simulink model "PMSM_Lq_Ke"  (R2024a)
settings: Solver=FixedStepAuto  StartTime=0.0  StopTime=0.5  FixedStep=1E-6  RelTol=1e-3
model workspace (MAT data in the model file):
  PWM_Frequency = Simulink.Parameter
  PWM_Frequency.Value = 30000
  PWM_Frequency.Complexity = 'real'
  PWM_Frequency.Dimensions = [1 1]
  PWM_Frequency.DataType = 'double'
  TimerPeriod = 0.1
values from neighbouring files (symbols this model uses):
  Flux = 0.01837    [Flux_Nonsensor_data_new.m]
undefined symbols (not defined in the file or in its folder): Down, Up
libraries: eePwmGenerator x4, slpidlib x3, spsDCVoltageSourceLib x1, spsPermanentMagnetSynchronousMachineLib x1, spsUniversalBridgeLib x1, sps_lib x1
settings Model: Creator=shish  LastModifiedBy=shish

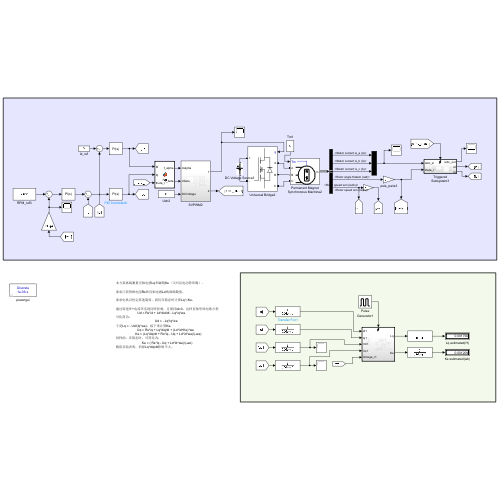
[thumbnail: Simulink's stored preview of the top-level diagram]
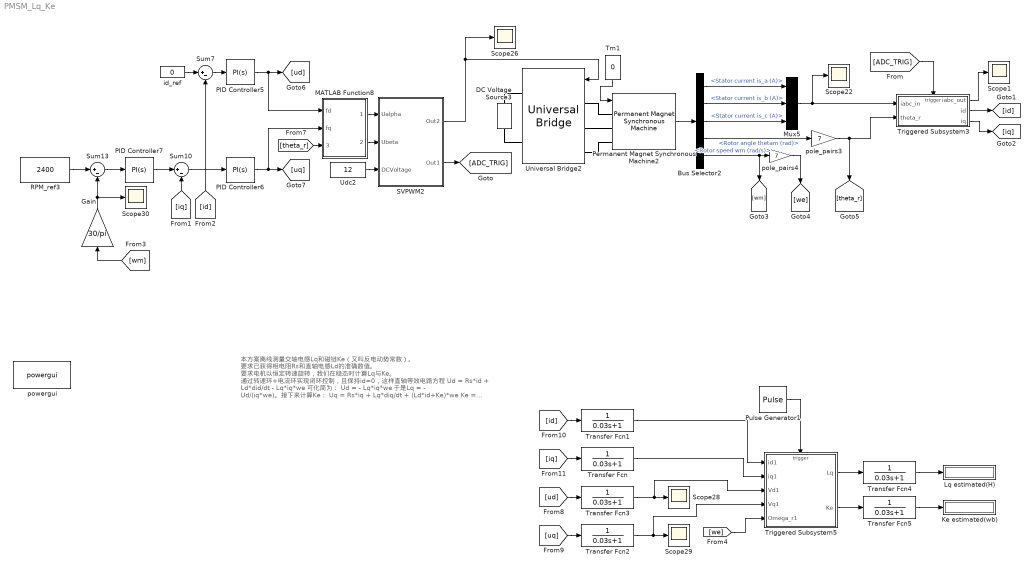
== system PMSM_Lq_Ke ==
  note: 本方案离线测量交轴电感Lq和磁链Ke（又叫反电动势常数）。
      |
      | 要求已获得相电阻Rs和直轴电感Ld的准确数值。
      |
      | 要求电机以恒定转速旋转，我们在稳态时计算Lq与Ke。
      |
      | 通过转速环+电流环实现闭环控制，且保持id=0，这样直轴等效电路方程
      |                         Ud = Rs*id + Ld*did/dt - Lq*iq*we
      | 可化简为：
      | 						Ud = - Lq*iq*we
      | 于是Lq = - Ud/(iq*we)。接下来计算Ke：
      | 			  Uq = Rs*iq + Lq*diq/dt + (Ld*id+Ke)*we
      | 			Ke = (Lq*diq/dt + Rs*iq - Uq + Ld*id*we)/(-we)
      | 同样的，在稳态时，可简化为：
      | 				Ke = ( Rs*iq - Uq + Ld*id*we)/(-we)
      | 数值实验表明，扔掉Lq*diq/dt影响不大。
  Bus Selector2 : BusSelector  OutputSignals=Stator current is_a (A),Stator current is_b (A),Stator current is_c (A),Rotor angle thetam (rad),Rotor speed wm (rad/s)
  DC Voltage Source3 : spsDCVoltageSourceLib/DC Voltage Source  Amplitude=12  Measurements=Voltage
  Gain : Gain  Gain=30/pi
  Ke estimated(wb) : Display
  Lq estimated(H) : Display
  MATLAB Function8 : MATLAB Function  TreatAsAtomicUnit=on
  Mux5 : Mux  Inputs=3
  PID Controller5 : slpidlib/PID Controller  Controller=PI  Form=Parallel  TimeDomain=Continuous-time  UseExternalTs=off  SampleTime=-1  IntegratorMethod=Forward Euler  FilterMethod=Forward Euler  ControllerParametersSource=internal  P=5  I=1  UseKiTs=on  D=0  UseExternalDerivativeSource=off  N=100  UseFilter=on  TunerSelectOption=Transfer Function Based (PID Tuner App)  InitialConditionSource=internal  InitialConditionForIntegrator=0  InitialConditionForFilter=0  DifferentiatorICPrevScaledInput=0  ExternalReset=none  TrackingMode=off  Kt=1  LimitOutput=off  SatLimitsSource=internal  UpperSaturationLimit=inf  LowerSaturationLimit=-inf  LinearizeAsGain=on  AntiWindupMode=none  Kb=1  LimitIntegrator=off  UpperIntegratorSaturationLimit=inf  LowerIntegratorSaturationLimit=-inf  POutMin=[]  POutMax=[]  IOutMin=[]  IOutMax=[]  DOutMin=[]  DOutMax=[]  NOutMin=[]  NOutMax=[]  SumOutMin=[]  SumOutMax=[]  SaturationOutMin=[]  SaturationOutMax=[]  PParamMin=[]  PParamMax=[]  IParamMin=[]  IParamMax=[]  DParamMin=[]  DParamMax=[]  NParamMin=[]  NParamMax=[]  KbParamMin=[]  KbParamMax=[]  KtParamMin=[]  KtParamMax=[]  KbOutMin=[]  KbOutMax=[]  KtOutMin=[]  KtOutMax=[]  IntegratorOutMin=[]  IntegratorOutMax=[]  FilterOutMin=[]  FilterOutMax=[]  SumI1OutMin=[]  SumI1OutMax=[]  SumI2OutMin=[]  SumI2OutMax=[]  SumI3OutMin=[]  SumI3OutMax=[]  SumI4OutMin=[]  SumI4OutMax=[]  SumDOutMin=[]  SumDOutMax=[]  DifferentiatorOutMin=[]  DifferentiatorOutMax=[]  FilterDiffOutCoefMin=[]  FilterDiffOutCoefMax=[]  ReciprocalOutMin=[]  ReciprocalOutMax=[]  SumDenOutMin=[]  SumDenOutMax=[]  SumNumOutMin=[]  SumNumOutMax=[]  DivideOutMin=[]  DivideOutMax=[]  UdiffTsProdOutMin=[]  UdiffTsProdOutMax=[]  NTsProdOutMin=[]  NTsProdOutMax=[]  UintegralTsProdOutMin=[]  UintegralTsProdOutMax=[]  UngainTsProdOutMin=[]  UngainTsProdOutMax=[]  ClampingZeroOutDataTypeStr=Inherit: Inherit via back propagation  ClampingZeroOutMin=[]  ClampingZeroOutMax=[]  FilterDenConstantOutDataTypeStr=Inherit: Inherit via back propagation  FilterDenConstantOutMin=[]  FilterDenConstantOutMax=[]  PCopyOutDataTypeStr=Inherit: Inherit via back propagation  PCopyOutMin=[]  PCopyOutMax=[]  NCopyOutDataTypeStr=Inherit: Inherit via back propagation  NCopyOutMin=[]  NCopyOutMax=[]  IntegratorContinuousStateAttributes=''  IntegratorStateMustResolveToSignalObject=off  IntegratorRTWStateStorageClass=Auto  FilterContinuousStateAttributes=''  FilterStateMustResolveToSignalObject=off  FilterRTWStateStorageClass=Auto  ParallelPVariant=InternalParameters  IdealPVariant=Disabled  IVariant=InternalParameters  DVariant=Disabled  IntegratorVariant=Continuous  SatVariant=Disabled  AWVariant=Passthrough  PCopyVariant=Disabled  TRVariant=Disabled  FdbkBlocksVariant=Forward  IdealPFdbkVariant=Disabled  SatFdbkVariant=Disabled  DerivativeFilterVariant=Disabled  NVariant=Disabled  NCopyVariant=Disabled_SignalSpec  FilterICVariant=Disabled  IntegratorICVariant=InternalICs  ExternalResetVariant=Disabled  TRSumVariant=Passthrough  SumFdbkVariant=Disabled  SumVariant=Sum_PI  TsampFilterVariant=InternalTs  TsampNgainVariant=Passthrough  TsampIntegralVariant=Disabled_SignalSpec  ExternalSaturationOutDataTypeStr=Inherit: Same as second input  DerivativeSourceVariant=Disabled
  PID Controller6 : slpidlib/PID Controller  Controller=PI  Form=Parallel  TimeDomain=Continuous-time  UseExternalTs=off  SampleTime=-1  IntegratorMethod=Forward Euler  FilterMethod=Forward Euler  ControllerParametersSource=internal  P=5  I=1  UseKiTs=on  D=0  UseExternalDerivativeSource=off  N=100  UseFilter=on  TunerSelectOption=Transfer Function Based (PID Tuner App)  InitialConditionSource=internal  InitialConditionForIntegrator=0  InitialConditionForFilter=0  DifferentiatorICPrevScaledInput=0  ExternalReset=none  TrackingMode=off  Kt=1  LimitOutput=off  SatLimitsSource=internal  UpperSaturationLimit=inf  LowerSaturationLimit=-inf  LinearizeAsGain=on  AntiWindupMode=none  Kb=1  LimitIntegrator=off  UpperIntegratorSaturationLimit=inf  LowerIntegratorSaturationLimit=-inf  POutMin=[]  POutMax=[]  IOutMin=[]  IOutMax=[]  DOutMin=[]  DOutMax=[]  NOutMin=[]  NOutMax=[]  SumOutMin=[]  SumOutMax=[]  SaturationOutMin=[]  SaturationOutMax=[]  PParamMin=[]  PParamMax=[]  IParamMin=[]  IParamMax=[]  DParamMin=[]  DParamMax=[]  NParamMin=[]  NParamMax=[]  KbParamMin=[]  KbParamMax=[]  KtParamMin=[]  KtParamMax=[]  KbOutMin=[]  KbOutMax=[]  KtOutMin=[]  KtOutMax=[]  IntegratorOutMin=[]  IntegratorOutMax=[]  FilterOutMin=[]  FilterOutMax=[]  SumI1OutMin=[]  SumI1OutMax=[]  SumI2OutMin=[]  SumI2OutMax=[]  SumI3OutMin=[]  SumI3OutMax=[]  SumI4OutMin=[]  SumI4OutMax=[]  SumDOutMin=[]  SumDOutMax=[]  DifferentiatorOutMin=[]  DifferentiatorOutMax=[]  FilterDiffOutCoefMin=[]  FilterDiffOutCoefMax=[]  ReciprocalOutMin=[]  ReciprocalOutMax=[]  SumDenOutMin=[]  SumDenOutMax=[]  SumNumOutMin=[]  SumNumOutMax=[]  DivideOutMin=[]  DivideOutMax=[]  UdiffTsProdOutMin=[]  UdiffTsProdOutMax=[]  NTsProdOutMin=[]  NTsProdOutMax=[]  UintegralTsProdOutMin=[]  UintegralTsProdOutMax=[]  UngainTsProdOutMin=[]  UngainTsProdOutMax=[]  ClampingZeroOutDataTypeStr=Inherit: Inherit via back propagation  ClampingZeroOutMin=[]  ClampingZeroOutMax=[]  FilterDenConstantOutDataTypeStr=Inherit: Inherit via back propagation  FilterDenConstantOutMin=[]  FilterDenConstantOutMax=[]  PCopyOutDataTypeStr=Inherit: Inherit via back propagation  PCopyOutMin=[]  PCopyOutMax=[]  NCopyOutDataTypeStr=Inherit: Inherit via back propagation  NCopyOutMin=[]  NCopyOutMax=[]  IntegratorContinuousStateAttributes=''  IntegratorStateMustResolveToSignalObject=off  IntegratorRTWStateStorageClass=Auto  FilterContinuousStateAttributes=''  FilterStateMustResolveToSignalObject=off  FilterRTWStateStorageClass=Auto  ParallelPVariant=InternalParameters  IdealPVariant=Disabled  IVariant=InternalParameters  DVariant=Disabled  IntegratorVariant=Continuous  SatVariant=Disabled  AWVariant=Passthrough  PCopyVariant=Disabled  TRVariant=Disabled  FdbkBlocksVariant=Forward  IdealPFdbkVariant=Disabled  SatFdbkVariant=Disabled  DerivativeFilterVariant=Disabled  NVariant=Disabled  NCopyVariant=Disabled_SignalSpec  FilterICVariant=Disabled  IntegratorICVariant=InternalICs  ExternalResetVariant=Disabled  TRSumVariant=Passthrough  SumFdbkVariant=Disabled  SumVariant=Sum_PI  TsampFilterVariant=InternalTs  TsampNgainVariant=Passthrough  TsampIntegralVariant=Disabled_SignalSpec  ExternalSaturationOutDataTypeStr=Inherit: Same as second input  DerivativeSourceVariant=Disabled
  PID Controller7 : slpidlib/PID Controller  Controller=PI  Form=Parallel  TimeDomain=Continuous-time  UseExternalTs=off  SampleTime=-1  IntegratorMethod=Forward Euler  FilterMethod=Forward Euler  ControllerParametersSource=internal  P=0.008  I=0.005  UseKiTs=on  D=0  UseExternalDerivativeSource=off  N=100  UseFilter=on  TunerSelectOption=Transfer Function Based (PID Tuner App)  InitialConditionSource=internal  InitialConditionForIntegrator=0  InitialConditionForFilter=0  DifferentiatorICPrevScaledInput=0  ExternalReset=none  TrackingMode=off  Kt=1  LimitOutput=off  SatLimitsSource=internal  UpperSaturationLimit=inf  LowerSaturationLimit=-inf  LinearizeAsGain=on  AntiWindupMode=none  Kb=1  LimitIntegrator=off  UpperIntegratorSaturationLimit=inf  LowerIntegratorSaturationLimit=-inf  POutMin=[]  POutMax=[]  IOutMin=[]  IOutMax=[]  DOutMin=[]  DOutMax=[]  NOutMin=[]  NOutMax=[]  SumOutMin=[]  SumOutMax=[]  SaturationOutMin=[]  SaturationOutMax=[]  PParamMin=[]  PParamMax=[]  IParamMin=[]  IParamMax=[]  DParamMin=[]  DParamMax=[]  NParamMin=[]  NParamMax=[]  KbParamMin=[]  KbParamMax=[]  KtParamMin=[]  KtParamMax=[]  KbOutMin=[]  KbOutMax=[]  KtOutMin=[]  KtOutMax=[]  IntegratorOutMin=[]  IntegratorOutMax=[]  FilterOutMin=[]  FilterOutMax=[]  SumI1OutMin=[]  SumI1OutMax=[]  SumI2OutMin=[]  SumI2OutMax=[]  SumI3OutMin=[]  SumI3OutMax=[]  SumI4OutMin=[]  SumI4OutMax=[]  SumDOutMin=[]  SumDOutMax=[]  DifferentiatorOutMin=[]  DifferentiatorOutMax=[]  FilterDiffOutCoefMin=[]  FilterDiffOutCoefMax=[]  ReciprocalOutMin=[]  ReciprocalOutMax=[]  SumDenOutMin=[]  SumDenOutMax=[]  SumNumOutMin=[]  SumNumOutMax=[]  DivideOutMin=[]  DivideOutMax=[]  UdiffTsProdOutMin=[]  UdiffTsProdOutMax=[]  NTsProdOutMin=[]  NTsProdOutMax=[]  UintegralTsProdOutMin=[]  UintegralTsProdOutMax=[]  UngainTsProdOutMin=[]  UngainTsProdOutMax=[]  ClampingZeroOutDataTypeStr=Inherit: Inherit via back propagation  ClampingZeroOutMin=[]  ClampingZeroOutMax=[]  FilterDenConstantOutDataTypeStr=Inherit: Inherit via back propagation  FilterDenConstantOutMin=[]  FilterDenConstantOutMax=[]  PCopyOutDataTypeStr=Inherit: Inherit via back propagation  PCopyOutMin=[]  PCopyOutMax=[]  NCopyOutDataTypeStr=Inherit: Inherit via back propagation  NCopyOutMin=[]  NCopyOutMax=[]  IntegratorContinuousStateAttributes=''  IntegratorStateMustResolveToSignalObject=off  IntegratorRTWStateStorageClass=Auto  FilterContinuousStateAttributes=''  FilterStateMustResolveToSignalObject=off  FilterRTWStateStorageClass=Auto  ParallelPVariant=InternalParameters  IdealPVariant=Disabled  IVariant=InternalParameters  DVariant=Disabled  IntegratorVariant=Continuous  SatVariant=Disabled  AWVariant=Passthrough  PCopyVariant=Disabled  TRVariant=Disabled  FdbkBlocksVariant=Forward  IdealPFdbkVariant=Disabled  SatFdbkVariant=Disabled  DerivativeFilterVariant=Disabled  NVariant=Disabled  NCopyVariant=Disabled_SignalSpec  FilterICVariant=Disabled  IntegratorICVariant=InternalICs  ExternalResetVariant=Disabled  TRSumVariant=Passthrough  SumFdbkVariant=Disabled  SumVariant=Sum_PI  TsampFilterVariant=InternalTs  TsampNgainVariant=Passthrough  TsampIntegralVariant=Disabled_SignalSpec  ExternalSaturationOutDataTypeStr=Inherit: Same as second input  DerivativeSourceVariant=Disabled
  Permanent Magnet Synchronous Machine2 : spsPermanentMagnetSynchronousMachineLib/Permanent Magnet Synchronous Machine  NbPhases=3  FluxDistribution=Sinusoidal  RotorType=Salient-pole  MechanicalLoad=Torque Tm  PresetModel=No  ShowDetailedParameters=on  MeasurementBus=off  Resistance=0.05  Inductance=8.5e-3  dqInductances=[1.8e-3,1.75e-3]  La=0.000395  MachineConstant=Flux linkage established by magnets (V.s)  Flux=0.0012  VoltageCst=1.5236  TorqueCst=0.0126  Flat=120  Mechanical=[0.000012 0.000005 7 0]  PolePairs=4  InitialConditions=[0,0, 0,0]  InitialConditions5ph=[0 0 0 0 0 0]  RefAngle=Aligned with phase A axis (original Park)  IterativeDiscreteModel=Trapezoidal non iterative  TsBlock=-1  TsPowergui=0
  Pulse Generator1 : DiscretePulseGenerator  PulseType=Time based  Period=0.005  PulseWidth=30
  RPM_ref3 : Constant  Value=2400
  SVPWM2 : Subsystem
  Scope{1,22,26,28..30} (6 alike) : Scope
  Sum10 : Sum  Inputs=|+-
  Sum13 : Sum  Inputs=|+-
  Sum7 : Sum  Inputs=|+-
  Tm1 : Constant  Value=0
  Transfer Fcn{,1..5} (6 alike) : TransferFcn  Denominator=[0.03 1]
  Triggered Subsystem3 : Subsystem  TreatAsAtomicUnit=on
  Triggered Subsystem5 : Subsystem  TreatAsAtomicUnit=on
  Udc2 : Constant  Value=12
  Universal Bridge2 : spsUniversalBridgeLib/Universal Bridge  Arms=3  SnubberResistance=1e5  SnubberCapacitance=inf  Device=MOSFET / Diodes  Ron=1e-3  Lon=0  ForwardVoltages="[  0  0  ]"  ForwardVoltage=0  GTOparameters=[ 10e-6 , 20e-6 ]  IGBTparameters=[ 1e-6 , 2e-6 ]  Measurements=None  Measurements_2=None  converterType=Rectifier
  id_ref : Constant  Value=0
  pole_pairs3 : Gain  Gain=7
  pole_pairs4 : Gain  Gain=7
  powergui : sps_lib/powergui  Priority=1  SimulationMode=Discrete  SampleTime=1e-6  frequency=60  Iterations=50  frequencyindice=0  Pbase=100e6  ErrMax=1e-4  UnitsV=kV  UnitsW=MW  buscounter=0  FunctionMessages=off  echomessages=off  EnableUseOfTLC=off  CurrentSourceSwitches=off  DisableSnubberDevices=off  DisableRonSwitches=off  DisableVfSwitches=off  DisplayEquations=off  AutomaticDiscreteSolvers=off  SolverType=Tustin/Backward Euler (TBE)  Interpol=off  ExternalGateDelay=off  methode=off  Ts=100  x0status=blocks  SPID=on  SwTol=0  HookPort=off  NonlinearTolerance=1e-4  nMaxIteration=100  ContinueOnMaxIteration=off  RestoreLinks=warning  ResistiveCurrentMeasurement=off  Frange=[0:2:500]  Ylog=off  Xlog=on  ShowGrid=off  save=off  variable=ZData  structure=0  ZoomFFT=off  StartTime=0.0  cycles=1  DisplayStyle=1  fundamental=60  FreqAxis=off  MaxFrequency=1000  frequencyindicesteady=1  RmsSteady=1  display=off
  wires:
  Bus Selector2/5 -> pole_pairs4/1, [wm]  "<Rotor speed wm (rad/s)>"
  MATLAB Function8/2(f_beta) -> SVPWM2/2(Ubeta)
  Bus Selector2/3 -> Mux5/3  "<Stator current is_c (A)>"
  MATLAB Function8/1(f_alpha) -> SVPWM2/1(Ualpha)
  Permanent Magnet Synchronous Machine2/1 -> Bus Selector2/1
  Bus Selector2/4 -> pole_pairs3/1  "<Rotor angle thetam (rad)>"
  Udc2/1 -> SVPWM2/3(DCVoltage)
  Bus Selector2/2 -> Mux5/2  "<Stator current is_b (A)>"
  Sum7/1 -> PID Controller5/1
  Sum10/1 -> PID Controller6/1
  PID Controller6/1 -> [uq], MATLAB Function8/2(fq)
  Mux5/1 -> Triggered Subsystem3/1(iabc_in), Scope22/1
  Tm1/1 -> Permanent Magnet Synchronous Machine2/1
  SVPWM2/1(Out2) -> Scope26/1, Universal Bridge2/1
  Bus Selector2/1 -> Mux5/1  "<Stator current is_a (A)>"
  id_ref/1 -> Sum7/1
  PID Controller5/1 -> [ud], MATLAB Function8/1(fd)
  Triggered Subsystem3/2(id) -> [id]
  Triggered Subsystem3/3(iq) -> [iq]
  pole_pairs4/1 -> [we]
  Transfer Fcn3/1 -> Triggered Subsystem5/3(Vd1), Scope28/1
  Transfer Fcn2/1 -> Triggered Subsystem5/4(Vq1), Scope29/1
  Gain/1 -> Scope30/1, Sum13/2
  Sum13/1 -> PID Controller7/1
  PID Controller7/1 -> Sum10/1
  Pulse Generator1/1 -> Triggered Subsystem5/Trigger
  SVPWM2/2(Out1) -> [ADC_TRIG]
  [ADC_TRIG] -> Triggered Subsystem3/Trigger
  [iq] -> Sum10/2
  [id] -> Sum7/2
  [wm] -> Gain/1
  [we] -> Triggered Subsystem5/5(Omega_r1)
  pole_pairs3/1 -> Triggered Subsystem3/2(theta_r), [theta_r]
  [theta_r] -> MATLAB Function8/3(theta_r)
  [ud] -> Transfer Fcn3/1
  [uq] -> Transfer Fcn2/1
  [id] -> Transfer Fcn1/1
  [iq] -> Transfer Fcn/1
  Transfer Fcn/1 -> Triggered Subsystem5/2(iq1)
  Transfer Fcn1/1 -> Triggered Subsystem5/1(id1)
  RPM_ref3/1 -> Sum13/1
  Triggered Subsystem5/1(Lq) -> Transfer Fcn4/1
  Triggered Subsystem5/2(Ke) -> Transfer Fcn5/1
  Transfer Fcn4/1 -> Lq estimated(H)/1
  Transfer Fcn5/1 -> Ke estimated(wb)/1
  Triggered Subsystem3/1(iabc_out) -> Scope1/1
  connections:
  Universal Bridge2/LConn2 -- Permanent Magnet Synchronous Machine2/LConn2
  Universal Bridge2/LConn1 -- Permanent Magnet Synchronous Machine2/LConn1
  DC Voltage Source3/LConn1 -- Universal Bridge2/RConn2
  DC Voltage Source3/RConn1 -- Universal Bridge2/RConn1
  Universal Bridge2/LConn3 -- Permanent Magnet Synchronous Machine2/LConn3

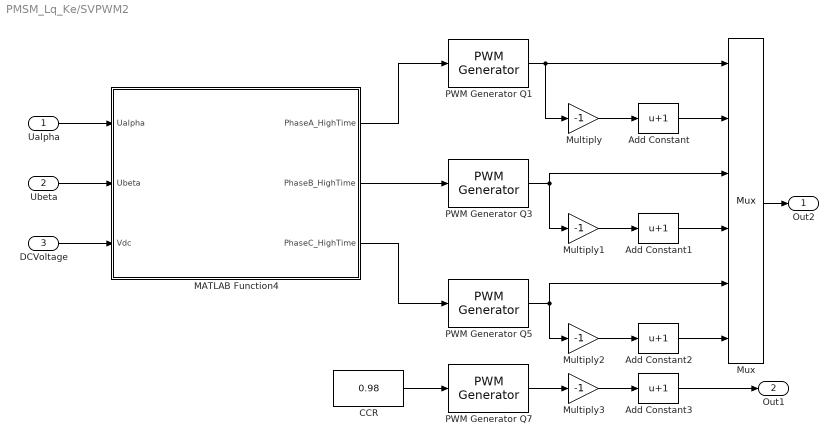
== system PMSM_Lq_Ke/SVPWM2 ==
  Ualpha : Inport
  Ubeta : Inport  Port=2
  DCVoltage : Inport  Port=3
  Add Constant{,1..3} (4 alike) : Bias  Bias=1  SaturateOnIntegerOverflow=off
  CCR : Constant  Value=0.98
  MATLAB Function4 : MATLAB Function  TreatAsAtomicUnit=on
  Multiply{,1..3} (4 alike) : Gain  Gain=-1
  Mux : Mux  Inputs=6
  PWM Generator Q{1,3,5,7} (4 alike) : eePwmGenerator/PWM Generator  CarrCount=Up-Down  Tper=1.0/PWM_Frequency  Tdelay=0  Ts=1E-6
  Out2 : Outport
  Out1 : Outport  Port=2
  wires:
  PWM Generator Q5/1 -> Mux/5, Multiply2/1
  PWM Generator Q1/1 -> Multiply/1, Mux/1
  Add Constant1/1 -> Mux/4
  Ubeta/1 -> MATLAB Function4/2(Ubeta)
  DCVoltage/1 -> MATLAB Function4/3(Vdc)
  MATLAB Function4/3(PhaseC_HighTime) -> PWM Generator Q5/1
  Multiply/1 -> Add Constant/1
  Multiply2/1 -> Add Constant2/1
  Add Constant/1 -> Mux/2
  MATLAB Function4/2(PhaseB_HighTime) -> PWM Generator Q3/1
  Add Constant2/1 -> Mux/6
  Multiply1/1 -> Add Constant1/1
  MATLAB Function4/1(PhaseA_HighTime) -> PWM Generator Q1/1
  Ualpha/1 -> MATLAB Function4/1(Ualpha)
  PWM Generator Q3/1 -> Mux/3, Multiply1/1
  PWM Generator Q7/1 -> Multiply3/1
  CCR/1 -> PWM Generator Q7/1
  Multiply3/1 -> Add Constant3/1
  Add Constant3/1 -> Out1/1
  Mux/1 -> Out2/1

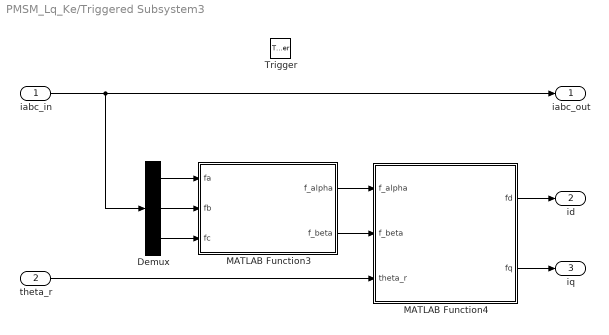
== system PMSM_Lq_Ke/Triggered Subsystem3 ==
  iabc_in : Inport
  theta_r : Inport  Port=2
  Trigger : TriggerPort  VariantControl=(inherit)
  Demux : Demux  Outputs=3
  MATLAB Function3 : MATLAB Function  TreatAsAtomicUnit=on
  MATLAB Function4 : MATLAB Function  TreatAsAtomicUnit=on
  iabc_out : Outport
  id : Outport  Port=2
  iq : Outport  Port=3
  wires:
  iabc_in/1 -> Demux/1, iabc_out/1
  Demux/3 -> MATLAB Function3/3(fc)
  Demux/2 -> MATLAB Function3/2(fb)
  Demux/1 -> MATLAB Function3/1(fa)
  MATLAB Function3/1(f_alpha) -> MATLAB Function4/1(f_alpha)
  MATLAB Function3/2(f_beta) -> MATLAB Function4/2(f_beta)
  theta_r/1 -> MATLAB Function4/3(theta_r)
  MATLAB Function4/1(fd) -> id/1
  MATLAB Function4/2(fq) -> iq/1

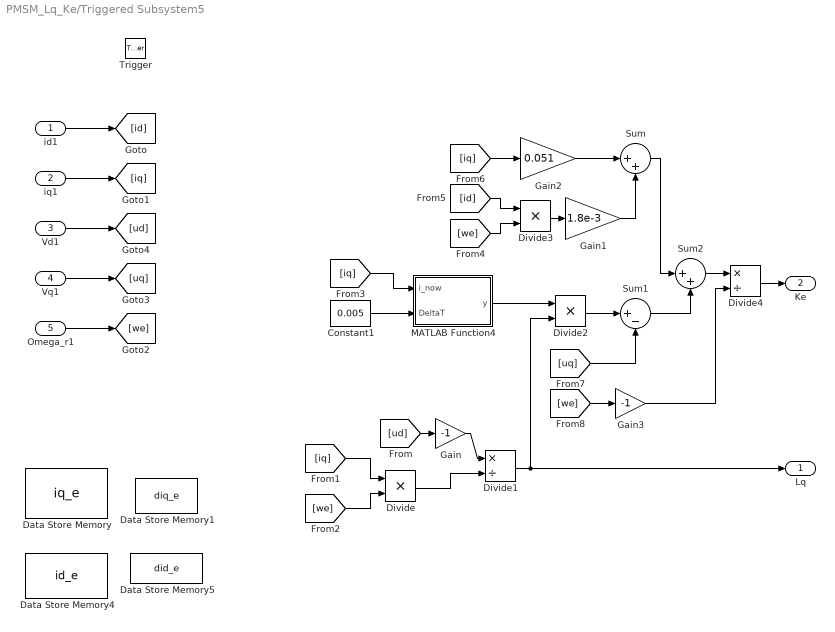
== system PMSM_Lq_Ke/Triggered Subsystem5 ==
  id1 : Inport
  iq1 : Inport  Port=2
  Vd1 : Inport  Port=3
  Vq1 : Inport  Port=4
  Omega_r1 : Inport  Port=5
  Trigger : TriggerPort  VariantControl=(inherit)
  Constant1 : Constant  Value=0.005
  Data Store Memory : DataStoreMemory  DataStoreName=iq_e  WriteAfterWriteMsg=warning  ShowAdditionalParam=off  OutDataTypeStr=double
  Data Store Memory1 : DataStoreMemory  DataStoreName=diq_e  WriteAfterWriteMsg=warning  ShowAdditionalParam=off  OutDataTypeStr=double
  Data Store Memory4 : DataStoreMemory  DataStoreName=id_e  WriteAfterWriteMsg=warning  ShowAdditionalParam=off  OutDataTypeStr=double
  Data Store Memory5 : DataStoreMemory  DataStoreName=did_e  WriteAfterWriteMsg=warning  ShowAdditionalParam=off  OutDataTypeStr=double
  Divide : Product  Inputs=**
  Divide1 : Product  Inputs=*/
  Divide2 : Product  Inputs=**
  Divide3 : Product  Inputs=**
  Divide4 : Product  Inputs=*/
  Gain : Gain  Gain=-1
  Gain1 : Gain  Gain=1.8e-3
  Gain2 : Gain  Gain=0.051
  Gain3 : Gain  Gain=-1
  MATLAB Function4 : MATLAB Function  TreatAsAtomicUnit=on
  Sum : Sum  Inputs=|++
  Sum1 : Sum  Inputs=|+-
  Sum2 : Sum  Inputs=|++
  Lq : Outport
  Ke : Outport  Port=2
  wires:
  Vd1/1 -> [ud]
  Vq1/1 -> [uq]
  Omega_r1/1 -> [we]
  id1/1 -> [id]
  iq1/1 -> [iq]
  Gain/1 -> Divide1/1
  Divide/1 -> Divide1/2
  Divide1/1 -> Divide2/2, Lq/1
  [ud] -> Gain/1
  [iq] -> Divide/1
  [we] -> Divide/2
  [iq] -> MATLAB Function4/1(i_now)
  Constant1/1 -> MATLAB Function4/2(DeltaT)
  MATLAB Function4/1(y) -> Divide2/1
  [id] -> Divide3/1
  [we] -> Divide3/2
  Divide3/1 -> Gain1/1
  [iq] -> Gain2/1
  Gain2/1 -> Sum/1
  Gain1/1 -> Sum/2
  [uq] -> Sum1/2
  Sum/1 -> Sum2/1
  Sum1/1 -> Sum2/2
  Sum2/1 -> Divide4/1
  Divide4/1 -> Ke/1
  [we] -> Gain3/1
  Gain3/1 -> Divide4/2
  Divide2/1 -> Sum1/1

== matlab function PMSM_Lq_Ke/Triggered Subsystem5/MATLAB Function4 ==
  data: i_now input; y output; iq_e data_store_memory; diq_e data_store_memory; DeltaT input
function y = TD(i_now,DeltaT)
	global iq_e;
    global diq_e;
	x1k = iq_e;
	x2k = diq_e;

	factor = x2k*x2k/3000.0;
    if factor < 1.0
		factor = 1.0;
    end
    h = DeltaT;
	h0 = 20*h;
    r = 20/h;
	fh = fhan(x1k - i_now, x2k, r*factor, h0);
	
	
	x1k = x1k + h*x2k;
	x2k = x2k + h*fh;

	iq_e = x1k;
	diq_e = x2k;
	
	y = x2k;

end

function y = fsg(x,d)
 y = (sign(x+d) - sign(x-d))/2.0;
end

function y = fhan(x1,x2,r,h)
 	d = r*h*h;
	a0 = h*x2;
	y = x1 + a0;

	a1 = sqrt(d*(d+8*abs(y)));
	a2 = a0 + 0.5*sign(y)*(a1-d);

	temp1 = fsg(y,d);
	a = (a0+y)*temp1 + a2*(1-temp1);

	temp2 = fsg(a,d);
	ret = -r*((a/d)*temp2 + sign(a)*(1-temp2));
	y = ret;
end

== matlab function PMSM_Lq_Ke/MATLAB Function8 ==
  data: fd input; f_alpha output; fq input; theta_r input; f_beta output
function [f_alpha,f_beta]= fcn(fd,fq,theta_r)
c = cos(theta_r);
s = sin(theta_r);
f_alpha =  c*fd - s*fq;
f_beta =  s*fd + c*fq;

== matlab function PMSM_Lq_Ke/SVPWM2/MATLAB Function4 ==
  data: Ualpha input; PhaseA_HighTime output; Ubeta input; Vdc input; PhaseB_HighTime output; PhaseC_HighTime output
function [PhaseA_HighTime,PhaseB_HighTime,PhaseC_HighTime] = SVPWM_calculate(Ualpha,Ubeta,Vdc)

% unit:V %

%step 1,which sector?%
if Ualpha >= 0
    %sector=1,2,5,6%
    if Ubeta >= 0
        %sector=1,2%
        if Ubeta > sqrt(3)*Ualpha
            sector=2;
        else
            sector=1;
        end
    else
        %sector=5,6%
        if -Ubeta > sqrt(3)*Ualpha
            sector=5;
        else
            sector=6;
        end
    end
else
    %sector=2,3,4,5%
    if Ubeta >= 0
        %sector=2,3%
        if Ubeta > -sqrt(3)*Ualpha
            sector=2;
        else
            sector=3;
        end
    else
        %sector=4,5%
        if -Ubeta > -sqrt(3)*Ualpha
            sector=5;
        else
            sector=4;
        end
    end
end

%step 2,vector decompose%
v1 = (2*Vdc/3)*[ 1,0];
v2 = (2*Vdc/3)*[ 0.5, 0.5*sqrt(3)];
v3 = (2*Vdc/3)*[-0.5, 0.5*sqrt(3)];
v4 = (2*Vdc/3)*[-1,0];
v5 = (2*Vdc/3)*[-0.5,-0.5*sqrt(3)];
v6 = (2*Vdc/3)*[ 0.5,-0.5*sqrt(3)];

if sector == 1
    vm=v1;vn=v2;
elseif sector == 2
    vm=v2;vn=v3;
elseif sector == 3
    vm=v3;vn=v4;
elseif sector == 4
    vm=v4;vn=v5;
elseif sector == 5
    vm=v5;vn=v6;
else
    vm=v6;vn=v1;
end

cm = (Ualpha*vn(2) - Ubeta*vn(1))/(vm(1)*vn(2) - vm(2)*vn(1));

if abs(vn(1))>1e-7
    cn = (Ualpha-cm*vm(1))/vn(1);
else
    cn = (Ubeta-cm*vm(2))/vn(2);
end
c_summ = cm+cn;
% if c_summ > 1
%     cm = cm/c_summ;
%     cn = cn/c_summ;
% end
if c_summ > 0.95
    cm = 0.95*cm/c_summ;
    cn = 0.95*cn/c_summ;
end

c0 = (1-cm-cn);
c0 = 0.5*c0;
c7 = c0;

%step 3,duty cycle%
if sector == 1
    %v1:100  v2:110%
    PhaseA_HighTime = cm+cn+c7;
    PhaseB_HighTime = cn+c7;
    PhaseC_HighTime = c7;
elseif sector == 2
    %v2:110  v3:010%
    PhaseA_HighTime = cm+c7;
    PhaseB_HighTime = cm+cn+c7;
    PhaseC_HighTime = c7;
elseif sector == 3
    %v3:010  v4:011%
    PhaseA_HighTime = c7;
    PhaseB_HighTime = cm+cn+c7;
    PhaseC_HighTime = cn+c7;
elseif sector == 4
    %v4:011  v5:001%
    PhaseA_HighTime = c7;
    PhaseB_HighTime = cm+c7;
    PhaseC_HighTime = cm+cn+c7;
elseif sector == 5
    %v5:001  v6:101%
    PhaseA_HighTime = cn+c7;
    PhaseB_HighTime = c7;
    PhaseC_HighTime = cm+cn+c7;
else
    %v6:101  v1:100%
    PhaseA_HighTime = cm+cn+c7;
    PhaseB_HighTime = c7;
    PhaseC_HighTime = cm+c7;
end

== matlab function PMSM_Lq_Ke/Triggered Subsystem3/MATLAB Function3 ==
  data: fa input; f_alpha output; fb input; fc input; f_beta output
function [f_alpha,f_beta]= ABC_to_AlphaBeta(fa,fb,fc)
f_alpha = (2/3)*(fa-0.5*(fb+fc));
f_beta = (2/3)*(0.5*sqrt(3)*(fb-fc));

== matlab function PMSM_Lq_Ke/Triggered Subsystem3/MATLAB Function4 ==
  data: f_alpha input; fd output; f_beta input; fq output; theta_r input
function [fd,fq]= AlphaBeta_to_dq(f_alpha,f_beta,theta_r)

c = cos(theta_r);
s = sin(theta_r);
fd =  c*f_alpha + s*f_beta;
fq = -s*f_alpha + c*f_beta;
